simulink model "complementary_filter"  (R2023b)
settings: Solver=FixedStepAuto  StartTime=0.0  StopTime=Tend_slk  FixedStep=Ts_slk  RelTol=1e-3
values from neighbouring files (symbols this model uses):
  acc_pole = 8    [complementary_filter_script.m]    (also in ekf2_script.m = 2)
  alpha = 0.95    [complementary_filter_script.m]
  P0_ps = 100    [complementary_filter_script.m]    (also in ekf1_script.m; ekf2_script.m; ekf3_script.m)
  q_ps = 100e-0    (= 100)    [complementary_filter_script.m]    (also in ekf1_script.m = 200; ekf2_script.m; ekf3_script.m = 170)
  r_ps = 600e+0    (= 600)    [complementary_filter_script.m]    (also in ekf1_script.m = 170; ekf2_script.m; ekf3_script.m = 200)
  Ts_EKF_integr = 0.001    [complementary_filter_script.m]    (also in ekf1_script.m = 0.0001; ekf2_script.m; ekf3_script.m = 0.0001)
  Ts_EKF_meas = 0.01    [complementary_filter_script.m]    (also in ekf1_script.m; ekf2_script.m; ekf3_script.m)
  Ts_meas = 0.01    [complementary_filter_script.m]
  Ts_slk = 0.01    [complementary_filter_script.m]    (also in ekf1_script.m; ekf2_script.m; ekf3_script.m)
  vel_pole = 30    [complementary_filter_script.m]    (also in ekf2_script.m = 20)
  x0_ps = 0    [complementary_filter_script.m]    (also in ekf2_script.m; ekf3_script.m)
settings Model: Creator=teoma  LastModifiedBy=teoma

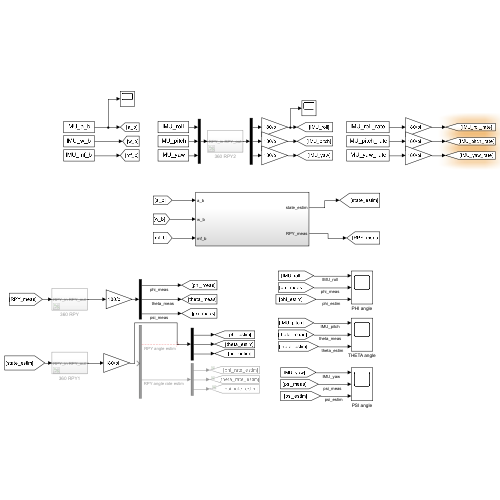
[thumbnail: Simulink's stored preview of the top-level diagram]
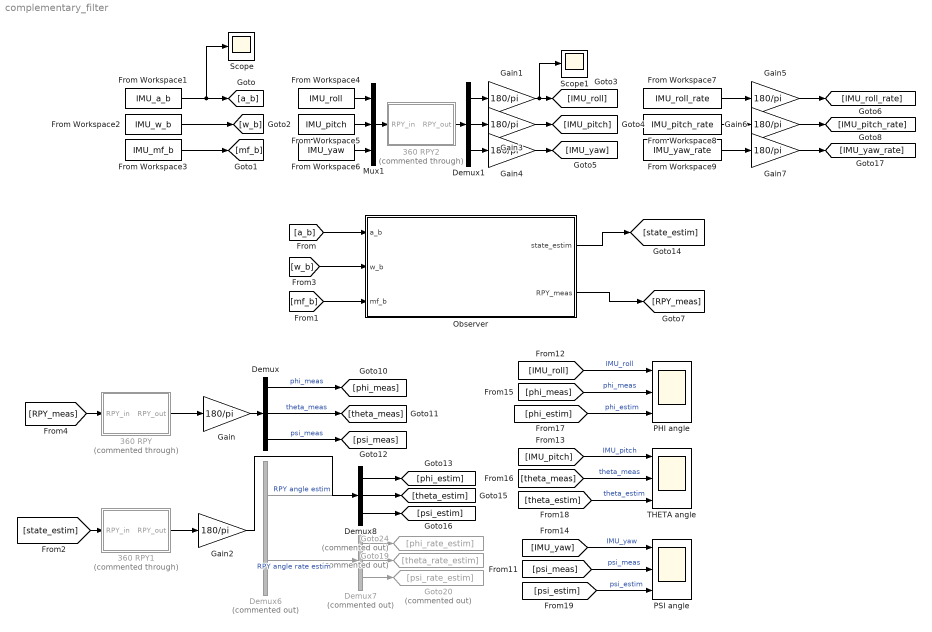
== system complementary_filter ==
  360 RPY : Subsystem  Commented=through
  360 RPY1 : Subsystem  Commented=through
  360 RPY2 : Subsystem  Commented=through
  Demux : Demux  Outputs=3
  Demux1 : Demux  Outputs=3
  Demux6 : Demux  Commented=on  Outputs=2
  Demux7 : Demux  Commented=on  Outputs=3
  Demux8 : Demux  Outputs=3
  From Workspace1 : FromWorkspace  VariableName=IMU_a_b  OutDataTypeStr=double  SampleTime=Ts_slk  Interpolate=off  OutputAfterFinalValue=Setting to zero
  From Workspace2 : FromWorkspace  VariableName=IMU_w_b  OutDataTypeStr=double  SampleTime=Ts_slk  Interpolate=off  OutputAfterFinalValue=Setting to zero
  From Workspace3 : FromWorkspace  VariableName=IMU_mf_b  OutDataTypeStr=double  SampleTime=Ts_slk  Interpolate=off  OutputAfterFinalValue=Setting to zero
  From Workspace4 : FromWorkspace  VariableName=IMU_roll  OutDataTypeStr=double  SampleTime=Ts_slk  Interpolate=off  OutputAfterFinalValue=Setting to zero
  From Workspace5 : FromWorkspace  VariableName=IMU_pitch  OutDataTypeStr=double  SampleTime=Ts_slk  Interpolate=off  OutputAfterFinalValue=Setting to zero
  From Workspace6 : FromWorkspace  VariableName=IMU_yaw  OutDataTypeStr=double  SampleTime=Ts_slk  Interpolate=off  OutputAfterFinalValue=Setting to zero
  From Workspace7 : FromWorkspace  VariableName=IMU_roll_rate  OutDataTypeStr=double  SampleTime=Ts_slk  Interpolate=off  OutputAfterFinalValue=Setting to zero
  From Workspace8 : FromWorkspace  VariableName=IMU_pitch_rate  OutDataTypeStr=double  SampleTime=Ts_slk  Interpolate=off  OutputAfterFinalValue=Setting to zero
  From Workspace9 : FromWorkspace  VariableName=IMU_yaw_rate  OutDataTypeStr=double  SampleTime=Ts_slk  Interpolate=off  OutputAfterFinalValue=Setting to zero
  Gain{,1..7} (8 alike) : Gain  Gain=180/pi
  Goto19 : Goto  Commented=on  GotoTag=theta_rate_estim
  Goto20 : Goto  Commented=on  GotoTag=psi_rate_estim
  Goto24 : Goto  Commented=on  GotoTag=phi_rate_estim
  Mux1 : Mux  Inputs=3
  Observer : Subsystem
  PHI angle : Scope  NumInputPorts=3
  PSI angle : Scope  NumInputPorts=3
  Scope : Scope
  Scope1 : Scope
  THETA angle : Scope  NumInputPorts=3
  wires:
  360 RPY2/1(RPY_out) -> Demux1/1
  From Workspace6/1 -> Mux1/3
  Demux1/3 -> Gain4/1
  Gain3/1 -> [IMU_pitch]
  Demux1/1 -> Gain1/1
  Demux1/2 -> Gain3/1
  From Workspace4/1 -> Mux1/1
  Gain6/1 -> [IMU_pitch_rate]
  From Workspace9/1 -> Gain7/1
  Gain5/1 -> [IMU_roll_rate]
  Mux1/1 -> 360 RPY2/1(RPY_in)
  From Workspace7/1 -> Gain5/1
  From Workspace8/1 -> Gain6/1
  From Workspace1/1 -> [a_b], Scope/1
  Gain1/1 -> Scope1/1, [IMU_roll]
  Gain7/1 -> [IMU_yaw_rate]
  Gain4/1 -> [IMU_yaw]
  From Workspace5/1 -> Mux1/2
  From Workspace3/1 -> [mf_b]
  From Workspace2/1 -> [w_b]
  Demux/2 -> [theta_meas]  "theta_meas"
  Demux7/1 -> Goto24/1
  Demux8/3 -> [psi_estim]
  [state_estim] -> 360 RPY1/1(RPY_in)
  Demux/3 -> [psi_meas]  "psi_meas"
  Demux7/3 -> Goto20/1
  Demux8/2 -> [theta_estim]
  [RPY_meas] -> 360 RPY/1(RPY_in)
  Demux6/1 -> ?  "RPY angle estim"
  [theta_estim] -> THETA angle/3  "theta_estim"
  [psi_estim] -> PSI angle/3  "psi_estim"
  Gain/1 -> Demux/1
  [IMU_pitch] -> THETA angle/1  "IMU_pitch"
  [phi_estim] -> PHI angle/3  "phi_estim"
  Demux/1 -> [phi_meas]  "phi_meas"
  [IMU_roll] -> PHI angle/1  "IMU_roll"
  Demux8/1 -> [phi_estim]
  Demux6/2 -> Demux7/1  "RPY angle rate estim"
  Demux7/2 -> Goto19/1
  Gain2/1 -> Demux8/1
  [psi_meas] -> PSI angle/2  "psi_meas"
  [theta_meas] -> THETA angle/2  "theta_meas"
  360 RPY/1(RPY_out) -> Gain/1
  [IMU_yaw] -> PSI angle/1  "IMU_yaw"
  [phi_meas] -> PHI angle/2  "phi_meas"
  360 RPY1/1(RPY_out) -> Gain2/1
  [mf_b] -> Observer/3(mf_b)
  [a_b] -> Observer/1(a_b)
  Observer/1(state_estim) -> [state_estim]
  Observer/2(RPY_meas) -> [RPY_meas]
  [w_b] -> Observer/2(w_b)

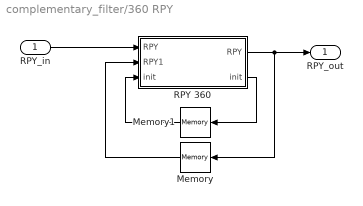
== system complementary_filter/360 RPY ==
  RPY_in : Inport
  Memory : Memory
  Memory1 : Memory
  RPY 360 : MATLAB Function  TreatAsAtomicUnit=on
  RPY_out : Outport
  wires:
  Memory/1 -> RPY 360/2(RPY1)
  Memory1/1 -> RPY 360/3("init ")
  RPY 360/2(init) -> Memory1/1
  RPY 360/1(RPY) -> Memory/1, RPY_out/1
  RPY_in/1 -> RPY 360/1("RPY ")

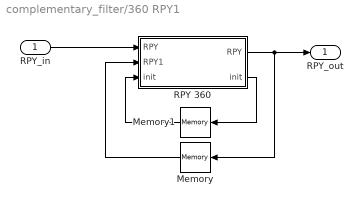
== system complementary_filter/360 RPY1 ==
  RPY_in : Inport
  Memory : Memory
  Memory1 : Memory
  RPY 360 : MATLAB Function  TreatAsAtomicUnit=on
  RPY_out : Outport
  wires:
  Memory/1 -> RPY 360/2(RPY1)
  Memory1/1 -> RPY 360/3("init ")
  RPY 360/2(init) -> Memory1/1
  RPY 360/1(RPY) -> Memory/1, RPY_out/1
  RPY_in/1 -> RPY 360/1("RPY ")

== system complementary_filter/360 RPY2 ==
  RPY_in : Inport
  Memory : Memory
  Memory1 : Memory
  RPY 360 : MATLAB Function  TreatAsAtomicUnit=on
  RPY_out : Outport
  wires:
  Memory/1 -> RPY 360/2(RPY1)
  Memory1/1 -> RPY 360/3("init ")
  RPY 360/2(init) -> Memory1/1
  RPY 360/1(RPY) -> Memory/1, RPY_out/1
  RPY_in/1 -> RPY 360/1("RPY ")

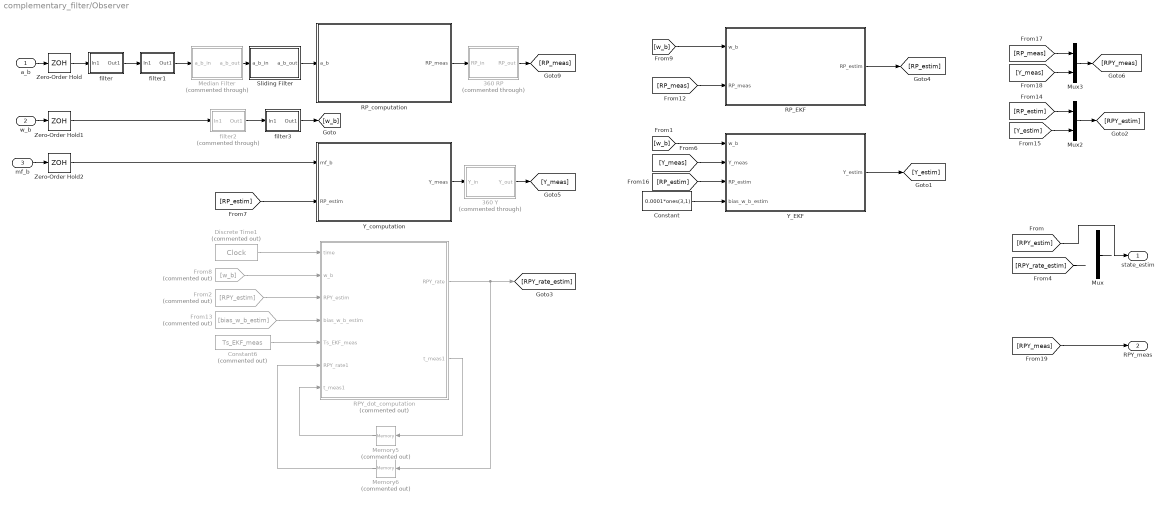
== system complementary_filter/Observer ==
  a_b : Inport
  w_b : Inport  Port=2
  mf_b : Inport  Port=3
  " filter" : Subsystem  mask{p=acc_pole}
      mask prompts: p "pole (p)"
  " filter1" : Subsystem  mask{p=acc_pole}
      mask prompts: p "pole (p)"
  " filter2" : Subsystem  Commented=through  mask{p=5}
      mask prompts: p "pole (p)"
  " filter3" : Subsystem  mask{p=vel_pole}
      mask prompts: p "pole (p)"
  360 RP : Subsystem  Commented=through
  360 Y : Subsystem  Commented=through
  Constant : Constant  Value=0.0001*ones(3,1)
  Constant6 : Constant  Commented=on  Value=Ts_EKF_meas
  Discrete Time1 : DigitalClock  Commented=on  SampleTime=Ts_slk
  From13 : From  Commented=on  GotoTag=bias_w_b_estim
  From2 : From  Commented=on  GotoTag=RPY_estim
  From8 : From  Commented=on  GotoTag=w_b
  Median Filter : Subsystem  Commented=through
  Memory5 : Memory  Commented=on
  Memory6 : Memory  Commented=on
  Mux : Mux  Inputs=2
  Mux2 : Mux  Inputs=2
  Mux3 : Mux  Inputs=2
  RPY_dot_computation : MATLAB Function  Commented=on  TreatAsAtomicUnit=on
  RP_EKF : Subsystem
  RP_computation : MATLAB Function  TreatAsAtomicUnit=on
  Sliding Filter : Subsystem
  Y_EKF : Subsystem
  Y_computation : MATLAB Function  TreatAsAtomicUnit=on
  Zero-Order Hold : ZeroOrderHold  SampleTime=Ts_meas
  Zero-Order Hold1 : ZeroOrderHold  SampleTime=Ts_meas
  Zero-Order Hold2 : ZeroOrderHold  SampleTime=Ts_meas
  state_estim : Outport
  RPY_meas : Outport  Port=2
  wires:
  Memory5/1 -> RPY_dot_computation/7("t_meas1 ")
  Discrete Time1/1 -> RPY_dot_computation/1(time)
  RPY_dot_computation/2(t_meas1) -> Memory5/1
  From8/1 -> RPY_dot_computation/2(w_b)
  Memory6/1 -> RPY_dot_computation/6(RPY_rate1)
  RPY_dot_computation/1(RPY_rate) -> Memory6/1, [RPY_rate_estim]
  Constant6/1 -> RPY_dot_computation/5(Ts_EKF_meas)
  From2/1 -> RPY_dot_computation/3(RPY_estim)
  From13/1 -> RPY_dot_computation/4(bias_w_b_estim)
  [RPY_estim] -> state_estim/1
  [RPY_rate_estim] -> ?
  Mux/1 -> ?
  [RPY_meas] -> RPY_meas/1
  [RP_estim] -> Y_computation/2(RP_estim)
  [Y_meas] -> Y_EKF/2(Y_meas)
  Y_computation/1(Y_meas) -> 360 Y/1(Y_in)
  RP_EKF/1(RP_estim) -> [RP_estim]
  [w_b] -> Y_EKF/1(w_b)
  RP_computation/1(RP_meas) -> 360 RP/1(RP_in)
  [RP_meas] -> RP_EKF/2(RP_meas)
  [w_b] -> RP_EKF/1(w_b)
  Y_EKF/1(Y_estim) -> [Y_estim]
  mf_b/1 -> Zero-Order Hold2/1
  w_b/1 -> Zero-Order Hold1/1
  Constant/1 -> Y_EKF/4(bias_w_b_estim)
  [RP_estim] -> Mux2/1
  [Y_estim] -> Mux2/2
  Mux2/1 -> [RPY_estim]
  [RP_estim] -> Y_EKF/3(RP_estim)
  [RP_meas] -> Mux3/1
  Mux3/1 -> [RPY_meas]
  [Y_meas] -> Mux3/2
  a_b/1 -> Zero-Order Hold/1
  " filter1"/1(Out1) -> Median Filter/1(a_b_in)
  360 Y/1(Y_out) -> [Y_meas]
  " filter"/1(Out1) -> " filter1"/1(In1)
  " filter2"/1(Out1) -> " filter3"/1(In1)
  " filter3"/1(Out1) -> [w_b]
  360 RP/1(RP_out) -> [RP_meas]
  Sliding Filter/1(a_b_out) -> RP_computation/1(a_b)
  Median Filter/1(a_b_out) -> Sliding Filter/1(a_b_in)
  Zero-Order Hold/1 -> " filter"/1(In1)
  Zero-Order Hold1/1 -> " filter2"/1(In1)
  Zero-Order Hold2/1 -> Y_computation/1(mf_b)

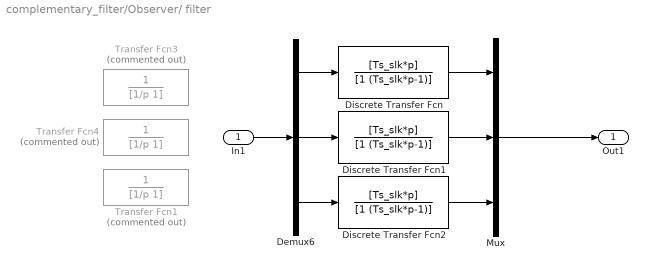
== system complementary_filter/Observer/ filter ==
  In1 : Inport
  Demux6 : Demux  Outputs=3
  Discrete Transfer Fcn : DiscreteTransferFcn  Numerator=[Ts_slk*p]  Denominator=[1 (Ts_slk*p-1)]
  Discrete Transfer Fcn1 : DiscreteTransferFcn  Numerator=[Ts_slk*p]  Denominator=[1 (Ts_slk*p-1)]
  Discrete Transfer Fcn2 : DiscreteTransferFcn  Numerator=[Ts_slk*p]  Denominator=[1 (Ts_slk*p-1)]
  Mux : Mux  Inputs=3
  Transfer Fcn1 : TransferFcn  Commented=on  Denominator=[1/p 1]
  Transfer Fcn3 : TransferFcn  Commented=on  Denominator=[1/p 1]
  Transfer Fcn4 : TransferFcn  Commented=on  Denominator=[1/p 1]
  Out1 : Outport
  wires:
  Discrete Transfer Fcn1/1 -> Mux/2
  Demux6/3 -> Discrete Transfer Fcn2/1
  Mux/1 -> Out1/1
  Discrete Transfer Fcn2/1 -> Mux/3
  Discrete Transfer Fcn/1 -> Mux/1
  In1/1 -> Demux6/1
  Demux6/1 -> Discrete Transfer Fcn/1
  Demux6/2 -> Discrete Transfer Fcn1/1

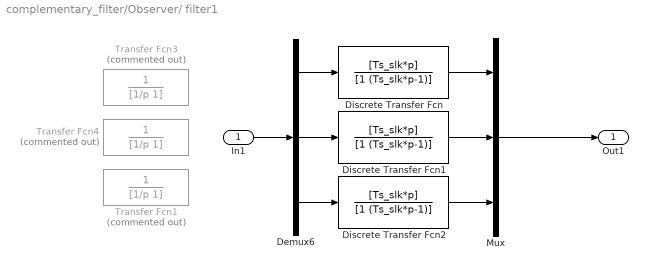
== system complementary_filter/Observer/ filter1 ==
  In1 : Inport
  Demux6 : Demux  Outputs=3
  Discrete Transfer Fcn : DiscreteTransferFcn  Numerator=[Ts_slk*p]  Denominator=[1 (Ts_slk*p-1)]
  Discrete Transfer Fcn1 : DiscreteTransferFcn  Numerator=[Ts_slk*p]  Denominator=[1 (Ts_slk*p-1)]
  Discrete Transfer Fcn2 : DiscreteTransferFcn  Numerator=[Ts_slk*p]  Denominator=[1 (Ts_slk*p-1)]
  Mux : Mux  Inputs=3
  Transfer Fcn1 : TransferFcn  Commented=on  Denominator=[1/p 1]
  Transfer Fcn3 : TransferFcn  Commented=on  Denominator=[1/p 1]
  Transfer Fcn4 : TransferFcn  Commented=on  Denominator=[1/p 1]
  Out1 : Outport
  wires:
  Discrete Transfer Fcn1/1 -> Mux/2
  Demux6/3 -> Discrete Transfer Fcn2/1
  Mux/1 -> Out1/1
  Discrete Transfer Fcn2/1 -> Mux/3
  Discrete Transfer Fcn/1 -> Mux/1
  In1/1 -> Demux6/1
  Demux6/1 -> Discrete Transfer Fcn/1
  Demux6/2 -> Discrete Transfer Fcn1/1

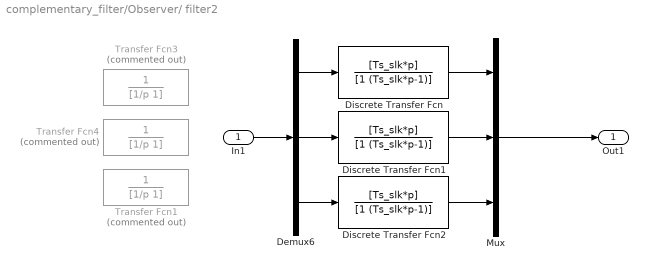
== system complementary_filter/Observer/ filter2 ==
  In1 : Inport
  Demux6 : Demux  Outputs=3
  Discrete Transfer Fcn : DiscreteTransferFcn  Numerator=[Ts_slk*p]  Denominator=[1 (Ts_slk*p-1)]
  Discrete Transfer Fcn1 : DiscreteTransferFcn  Numerator=[Ts_slk*p]  Denominator=[1 (Ts_slk*p-1)]
  Discrete Transfer Fcn2 : DiscreteTransferFcn  Numerator=[Ts_slk*p]  Denominator=[1 (Ts_slk*p-1)]
  Mux : Mux  Inputs=3
  Transfer Fcn1 : TransferFcn  Commented=on  Denominator=[1/p 1]
  Transfer Fcn3 : TransferFcn  Commented=on  Denominator=[1/p 1]
  Transfer Fcn4 : TransferFcn  Commented=on  Denominator=[1/p 1]
  Out1 : Outport
  wires:
  Discrete Transfer Fcn1/1 -> Mux/2
  Demux6/3 -> Discrete Transfer Fcn2/1
  Mux/1 -> Out1/1
  Discrete Transfer Fcn2/1 -> Mux/3
  Discrete Transfer Fcn/1 -> Mux/1
  In1/1 -> Demux6/1
  Demux6/1 -> Discrete Transfer Fcn/1
  Demux6/2 -> Discrete Transfer Fcn1/1

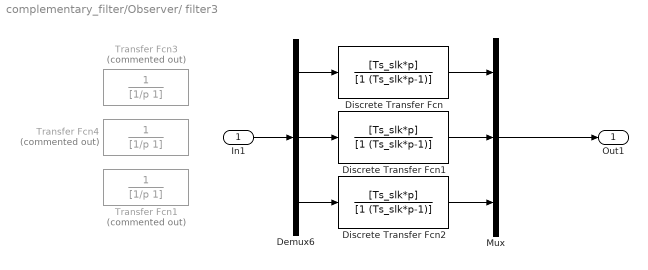
== system complementary_filter/Observer/ filter3 ==
  In1 : Inport
  Demux6 : Demux  Outputs=3
  Discrete Transfer Fcn : DiscreteTransferFcn  Numerator=[Ts_slk*p]  Denominator=[1 (Ts_slk*p-1)]
  Discrete Transfer Fcn1 : DiscreteTransferFcn  Numerator=[Ts_slk*p]  Denominator=[1 (Ts_slk*p-1)]
  Discrete Transfer Fcn2 : DiscreteTransferFcn  Numerator=[Ts_slk*p]  Denominator=[1 (Ts_slk*p-1)]
  Mux : Mux  Inputs=3
  Transfer Fcn1 : TransferFcn  Commented=on  Denominator=[1/p 1]
  Transfer Fcn3 : TransferFcn  Commented=on  Denominator=[1/p 1]
  Transfer Fcn4 : TransferFcn  Commented=on  Denominator=[1/p 1]
  Out1 : Outport
  wires:
  Discrete Transfer Fcn1/1 -> Mux/2
  Demux6/3 -> Discrete Transfer Fcn2/1
  Mux/1 -> Out1/1
  Discrete Transfer Fcn2/1 -> Mux/3
  Discrete Transfer Fcn/1 -> Mux/1
  In1/1 -> Demux6/1
  Demux6/1 -> Discrete Transfer Fcn/1
  Demux6/2 -> Discrete Transfer Fcn1/1

== system complementary_filter/Observer/360 RP ==
  RP_in : Inport
  Memory : Memory
  Memory1 : Memory
  RP 360 : MATLAB Function  TreatAsAtomicUnit=on
  RP_out : Outport
  wires:
  RP_in/1 -> RP 360/1("RP ")
  RP 360/1(RP) -> Memory/1, RP_out/1
  Memory/1 -> RP 360/2(RP1)
  RP 360/2(init) -> Memory1/1
  Memory1/1 -> RP 360/3("init ")

== system complementary_filter/Observer/360 Y ==
  Y_in : Inport
  Memory : Memory
  Memory1 : Memory
  Y 360 : MATLAB Function  TreatAsAtomicUnit=on
  Y_out : Outport
  wires:
  Y_in/1 -> Y 360/1("Y ")
  Y 360/1(Y) -> Memory/1, Y_out/1
  Memory/1 -> Y 360/2(Y1)
  Y 360/2(init) -> Memory1/1
  Memory1/1 -> Y 360/3("init ")

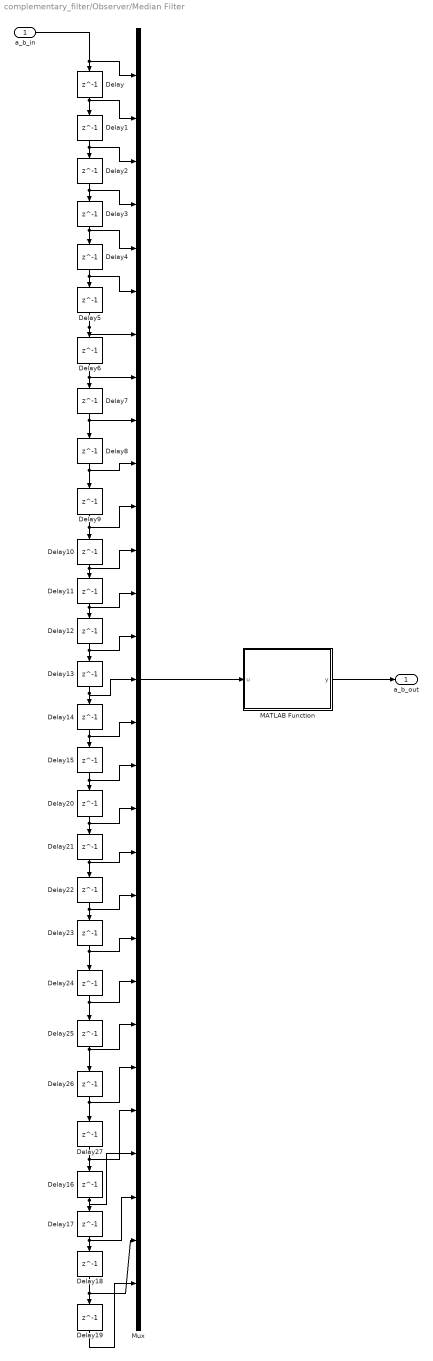
== system complementary_filter/Observer/Median Filter ==
  a_b_in : Inport
  Delay{,1..27} (28 alike) : Delay  DelayLength=1  InitialCondition=zeros(1,3)  SampleTime=Ts_slk
  MATLAB Function : MATLAB Function  TreatAsAtomicUnit=on
  Mux : Mux  Inputs=29
  a_b_out : Outport
  wires:
  a_b_in/1 -> Delay/1, Mux/1
  Delay1/1 -> Delay2/1, Mux/3
  Delay2/1 -> Delay3/1, Mux/4
  Delay/1 -> Delay1/1, Mux/2
  Delay3/1 -> Delay4/1, Mux/5
  Mux/1 -> MATLAB Function/1(u)
  MATLAB Function/1(y) -> a_b_out/1
  Delay4/1 -> Delay5/1, Mux/6
  Delay5/1 -> Delay6/1, Mux/7
  Delay6/1 -> Delay7/1, Mux/8
  Delay8/1 -> Mux/10, Delay9/1
  Delay11/1 -> Mux/13, Delay12/1
  Delay12/1 -> Mux/14, Delay13/1
  Delay7/1 -> Mux/9, Delay8/1
  Delay9/1 -> Delay10/1, Mux/11
  Delay10/1 -> Mux/12, Delay11/1
  Delay13/1 -> Mux/15, Delay14/1
  Delay24/1 -> Mux/22, Delay25/1
  Delay23/1 -> Mux/21, Delay24/1
  Delay20/1 -> Mux/18, Delay21/1
  Delay15/1 -> Mux/17, Delay20/1
  Delay21/1 -> Mux/19, Delay22/1
  Delay27/1 -> Mux/25, Delay16/1
  Delay18/1 -> Delay19/1, Mux/28
  Delay25/1 -> Mux/23, Delay26/1
  Delay22/1 -> Mux/20, Delay23/1
  Delay26/1 -> Mux/24, Delay27/1
  Delay14/1 -> Mux/16, Delay15/1
  Delay17/1 -> Mux/27, Delay18/1
  Delay16/1 -> Mux/26, Delay17/1
  Delay19/1 -> Mux/29

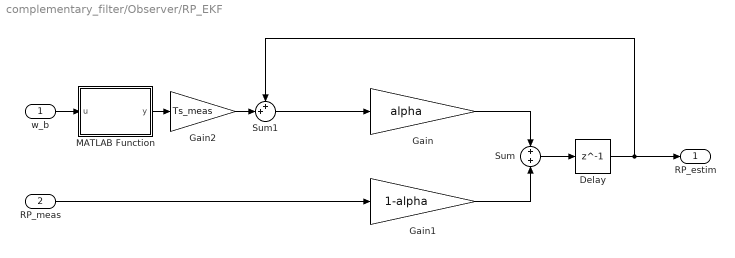
== system complementary_filter/Observer/RP_EKF ==
  w_b : Inport
  RP_meas : Inport  Port=2
  Delay : Delay  DelayLength=1  SampleTime=Ts_meas
  Gain : Gain  Gain=alpha
  Gain1 : Gain  Gain=1-alpha
  Gain2 : Gain  Gain=Ts_meas
  MATLAB Function : MATLAB Function  TreatAsAtomicUnit=on
  Sum : Sum  Inputs=+|+
  Sum1 : Sum  Inputs=++|
  RP_estim : Outport
  wires:
  w_b/1 -> MATLAB Function/1(u)
  RP_meas/1 -> Gain1/1
  MATLAB Function/1(y) -> Gain2/1
  Gain1/1 -> Sum/2
  Gain/1 -> Sum/1
  Sum/1 -> Delay/1
  Sum1/1 -> Gain/1
  Delay/1 -> RP_estim/1, Sum1/1
  Gain2/1 -> Sum1/2

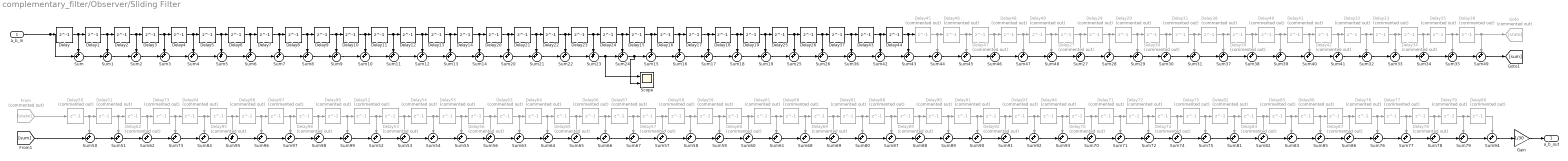
== system complementary_filter/Observer/Sliding Filter ==
  a_b_in : Inport
  Delay{,1..26,37,43..44} (30 alike) : Delay  DelayLength=1  SampleTime=Ts_meas
  Delay{27..36,38..42,45..99} (70 alike) : Delay  Commented=on  DelayLength=1  SampleTime=Ts_slk
  From : From  Commented=on  GotoTag=state
  Gain : Gain  Gain=1/30
  Goto : Goto  Commented=on  GotoTag=state
  Scope : Scope  NumInputPorts=2
  Sum{,1..99} (100 alike) : Sum  Inputs=++|
  a_b_out : Outport
  wires:
  Delay/1 -> Sum/1, Delay1/1
  Delay1/1 -> Sum1/1, Delay2/1
  Delay2/1 -> Sum2/1, Delay3/1
  Delay3/1 -> Sum3/1, Delay4/1
  Sum/1 -> Sum1/2
  Sum1/1 -> Sum2/2
  Sum2/1 -> Sum3/2
  Sum3/1 -> Sum4/2
  Delay4/1 -> Delay5/1, Sum4/1
  Sum4/1 -> Sum5/2
  a_b_in/1 -> Sum/2, Delay/1
  Delay5/1 -> Sum5/1, Delay6/1
  Delay6/1 -> Sum6/1, Delay7/1
  Sum5/1 -> Sum6/2
  Sum6/1 -> Sum7/2
  Sum7/1 -> Sum8/2
  Delay7/1 -> Sum7/1, Delay8/1
  Delay8/1 -> Delay9/1, Sum8/1
  Delay9/1 -> Sum9/1, Delay10/1
  Delay10/1 -> Sum10/1, Delay11/1
  Delay11/1 -> Sum11/1, Delay12/1
  Delay12/1 -> Sum12/1, Delay13/1
  Delay13/1 -> Sum13/1, Delay14/1
  Sum11/1 -> Sum12/2
  Sum12/1 -> Sum13/2
  Sum13/1 -> Sum14/2
  Sum8/1 -> Sum9/2
  Sum9/1 -> Sum10/2
  Sum10/1 -> Sum11/2
  Delay14/1 -> Delay20/1, Sum14/1
  Delay19/1 -> Delay25/1, Sum19/1
  Sum16/1 -> Sum17/2
  Delay15/1 -> Sum15/1, Delay16/1
  Sum24/1 -> Scope/2, Sum15/2
  Sum17/1 -> Sum18/2
  Delay23/1 -> Delay24/1, Sum23/1
  Delay24/1 -> Sum24/1, Delay15/1
  Sum20/1 -> Sum21/2
  Delay22/1 -> Sum22/1, Delay23/1
  Delay18/1 -> Sum18/1, Delay19/1
  Sum23/1 -> Scope/1, Sum24/2
  Sum22/1 -> Sum23/2
  Sum14/1 -> Sum20/2
  Delay20/1 -> Sum20/1, Delay21/1
  Delay17/1 -> Sum17/1, Delay18/1
  Sum18/1 -> Sum19/2
  Delay21/1 -> Sum21/1, Delay22/1
  Delay16/1 -> Sum16/1, Delay17/1
  Sum15/1 -> Sum16/2
  Sum21/1 -> Sum22/2
  Sum41/1 -> Sum32/2
  Delay32/1 -> Sum32/1, Delay33/1
  Sum33/1 -> Sum34/2
  Delay42/1 -> Sum41/1, Delay32/1
  Sum37/1 -> Sum38/2
  Delay41/1 -> Delay42/1, Sum40/1
  Delay31/1 -> Delay38/1, Sum31/1
  Sum28/1 -> Sum29/2
  Delay28/1 -> Sum28/1, Delay29/1
  Delay27/1 -> Sum27/1, Delay28/1
  Delay49/1 -> Sum48/1, Delay27/1
  Sum48/1 -> Sum27/2
  Sum29/1 -> Sum30/2
  Delay48/1 -> Delay49/1, Sum47/1
  Sum44/1 -> Sum45/2
  Delay47/1 -> Sum46/1, Delay48/1
  Delay45/1 -> Sum44/1, Delay46/1
  Delay39/1 -> Sum38/1, Delay40/1
  Sum47/1 -> Sum48/2
  Delay38/1 -> Sum37/1, Delay39/1
  Sum40/1 -> Sum41/2
  Sum46/1 -> Sum47/2
  Sum34/1 -> Sum35/2
  Delay29/1 -> Sum29/1, Delay30/1
  Sum32/1 -> Sum33/2
  Delay40/1 -> Sum39/1, Delay41/1
  Delay46/1 -> Sum45/1, Delay47/1
  Delay33/1 -> Sum33/1, Delay34/1
  Sum27/1 -> Sum28/2
  Delay30/1 -> Sum30/1, Delay31/1
  Sum36/1 -> Sum42/2
  Delay44/1 -> Delay45/1, Sum43/1
  Sum39/1 -> Sum40/2
  Delay37/1 -> Sum36/1, Delay43/1
  Sum26/1 -> Sum36/2
  Sum43/1 -> Sum44/2
  Sum25/1 -> Sum26/2
  Delay35/1 -> Sum35/1, Delay36/1
  Sum42/1 -> Sum43/2
  Delay43/1 -> Sum42/1, Delay44/1
  Sum30/1 -> Sum31/2
  Sum45/1 -> Sum46/2
  Sum31/1 -> Sum37/2
  Delay26/1 -> Sum26/1, Delay37/1
  Delay25/1 -> Sum25/1, Delay26/1
  Delay34/1 -> Sum34/1, Delay35/1
  Sum38/1 -> Sum39/2
  Sum35/1 -> Sum49/2
  Sum19/1 -> Sum25/2
  Delay36/1 -> Goto/1, Sum49/1
  Sum49/1 -> [sum]
  Delay68/1 -> Sum68/1, Delay69/1
  Sum82/1 -> Sum83/2
  Sum68/1 -> Sum69/2
  Sum75/1 -> Sum81/2
  Delay88/1 -> Sum87/1, Delay89/1
  Delay79/1 -> Sum79/1, Delay80/1
  Sum74/1 -> Sum75/2
  Delay69/1 -> Sum69/1, Delay81/1
  Sum90/1 -> Sum91/2
  Sum83/1 -> Sum85/2
  Sum80/1 -> Sum87/2
  Sum88/1 -> Sum89/2
  Sum69/1 -> Sum80/2
  Sum70/1 -> Sum71/2
  Delay78/1 -> Sum78/1, Delay79/1
  Sum92/1 -> Sum93/2
  Sum78/1 -> Sum79/2
  Sum91/1 -> Sum92/2
  Sum85/1 -> Sum86/2
  Sum76/1 -> Sum77/2
  Delay72/1 -> Sum72/1, Delay74/1
  Delay82/1 -> Sum81/1, Delay83/1
  Sum72/1 -> Sum74/2
  Delay94/1 -> Sum93/1, Delay70/1
  Delay85/1 -> Sum83/1, Delay86/1
  Delay74/1 -> Sum74/1, Delay75/1
  Sum93/1 -> Sum70/2
  Delay90/1 -> Sum89/1, Delay91/1
  Delay92/1 -> Sum91/1, Delay93/1
  Delay93/1 -> Delay94/1, Sum92/1
  Delay75/1 -> Delay82/1, Sum75/1
  Sum71/1 -> Sum72/2
  Delay71/1 -> Sum71/1, Delay72/1
  Delay70/1 -> Sum70/1, Delay71/1
  Sum67/1 -> Sum57/2
  Delay57/1 -> Sum57/1, Delay58/1
  Sum58/1 -> Sum59/2
  Sum89/1 -> Sum90/2
  Delay61/1 -> Delay68/1, Sum61/1
  Delay67/1 -> Sum67/1, Delay57/1
  Sum63/1 -> Sum64/2
  Delay66/1 -> Delay67/1, Sum66/1
  Sum94/1 -> Gain/1
  Sum81/1 -> Sum82/2
  Sum77/1 -> Sum78/2
  Delay87/1 -> Sum86/1, Delay76/1
  Delay76/1 -> Sum76/1, Delay77/1
  Delay86/1 -> Delay87/1, Sum85/1
  Sum86/1 -> Sum76/2
  Sum53/1 -> Sum54/2
  Delay53/1 -> Sum53/1, Delay54/1
  Delay56/1 -> Delay63/1, Sum56/1
  Delay52/1 -> Sum52/1, Delay53/1
  Delay99/1 -> Sum99/1, Delay52/1
  Sum99/1 -> Sum52/2
  Sum54/1 -> Sum55/2
  Delay98/1 -> Delay99/1, Sum98/1
  Sum95/1 -> Sum96/2
  Delay97/1 -> Sum97/1, Delay98/1
  Delay95/1 -> Sum95/1, Delay96/1
  Delay55/1 -> Sum55/1, Delay56/1
  Sum98/1 -> Sum99/2
  Sum64/1 -> Sum65/2
  Delay64/1 -> Sum64/1, Delay65/1
  Delay58/1 -> Sum58/1, Delay59/1
  Delay81/1 -> Sum80/1, Delay88/1
  Delay63/1 -> Sum63/1, Delay64/1
  Sum66/1 -> Sum67/2
  Sum97/1 -> Sum98/2
  Delay77/1 -> Sum77/1, Delay78/1
  Sum59/1 -> Sum60/2
  Delay54/1 -> Sum54/1, Delay55/1
  Sum57/1 -> Sum58/2
  Delay89/1 -> Delay90/1, Sum88/1
  Delay65/1 -> Sum65/1, Delay66/1
  Delay96/1 -> Sum96/1, Delay97/1
  Sum52/1 -> Sum53/2
  From/1 -> Delay50/1
  Delay83/1 -> Sum82/1, Delay85/1
  Sum62/1 -> Sum73/2
  Delay84/1 -> Delay95/1, Sum84/1
  Sum65/1 -> Sum66/2
  Sum87/1 -> Sum88/2
  Delay62/1 -> Sum62/1, Delay73/1
  Sum51/1 -> Sum62/2
  Delay91/1 -> Sum90/1, Delay92/1
  Sum84/1 -> Sum95/2
  Sum50/1 -> Sum51/2
  Delay60/1 -> Sum60/1, Delay61/1
  Sum73/1 -> Sum84/2
  Delay73/1 -> Sum73/1, Delay84/1
  Sum55/1 -> Sum56/2
  Sum61/1 -> Sum68/2
  Delay80/1 -> Sum94/1
  Sum96/1 -> Sum97/2
  Sum79/1 -> Sum94/2
  Sum56/1 -> Sum63/2
  Delay51/1 -> Sum51/1, Delay62/1
  Delay50/1 -> Sum50/1, Delay51/1
  Delay59/1 -> Sum59/1, Delay60/1
  Sum60/1 -> Sum61/2
  Gain/1 -> a_b_out/1
  [sum] -> Sum50/2

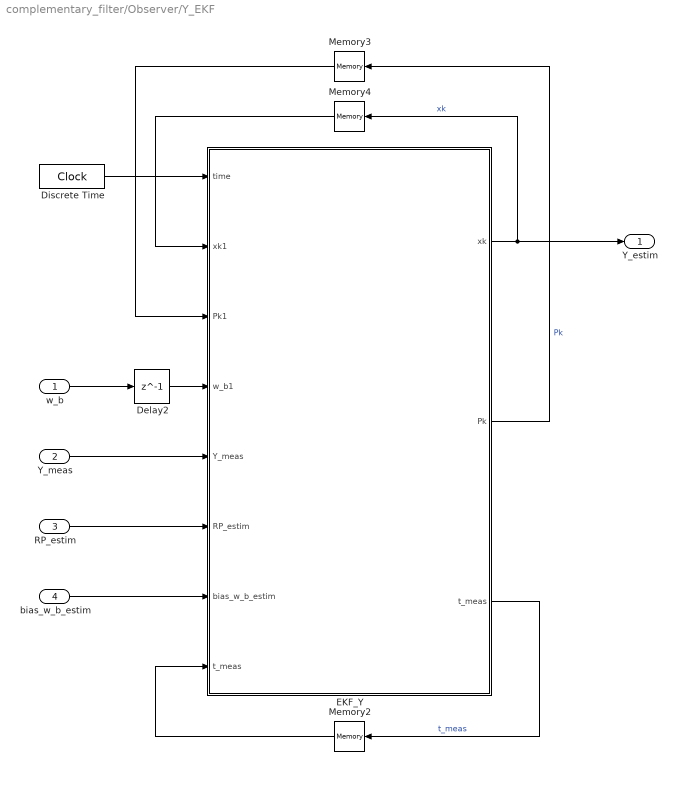
== system complementary_filter/Observer/Y_EKF ==
  w_b : Inport
  Y_meas : Inport  Port=2
  RP_estim : Inport  Port=3
  bias_w_b_estim : Inport  Port=4
  Delay2 : Delay  DelayLength=1  SampleTime=Ts_EKF_meas
  Discrete Time : DigitalClock  SampleTime=Ts_EKF_meas
  EKF_Y : MATLAB Function  TreatAsAtomicUnit=on
  Memory2 : Memory
  Memory3 : Memory  InitialCondition=ones(1,1)*P0_ps
  Memory4 : Memory  InitialCondition=ones(1,1)*x0_ps
  Y_estim : Outport
  wires:
  w_b/1 -> Delay2/1
  EKF_Y/2(Pk) -> Memory3/1  "Pk"
  Memory2/1 -> EKF_Y/8("t_meas ")
  EKF_Y/3(t_meas) -> Memory2/1  "t_meas"
  Y_meas/1 -> EKF_Y/5(Y_meas)
  Discrete Time/1 -> EKF_Y/1(time)
  Memory3/1 -> EKF_Y/3(Pk1)
  Delay2/1 -> EKF_Y/4(w_b1)
  Memory4/1 -> EKF_Y/2(xk1)
  EKF_Y/1(xk) -> Memory4/1, Y_estim/1  "xk"
  bias_w_b_estim/1 -> EKF_Y/7(bias_w_b_estim)
  RP_estim/1 -> EKF_Y/6(RP_estim)

== matlab function complementary_filter/360 RPY/RPY 360 ==
  data: RPY input; RPY output; RPY1 input; init output; init input
function [RPY,init] = RPY_360(RPY,RPY1,init)
if init < 2 
    if init == 0
        init = 1;
        RPY1 = RPY;
    elseif init == 1
        if (RPY - RPY1)'*(RPY - RPY1) > 0.01
            init = 2;
            RPY1 = RPY;
        end
    end
end

% - pi <= PHI <= + pi PHI uses atan2()
if abs(RPY(1) - RPY1(1)) > pi*0.99
    RPY(1) = RPY(1) + sign(RPY1(1))*(2*pi);
end
% - pi/2 <= THETA <= + pi/2 THETA uses asin()
if abs(RPY(2) - RPY1(2)) > pi/2*0.99
    RPY(2) = RPY(2) + sign(RPY1(2))*(2*pi);
end
% - pi <= PSI <= + pi PSI uses atan2()
if abs(RPY(3) - RPY1(3)) > pi*0.99
    RPY(3) = RPY(3) + sign(RPY1(3))*(2*pi);
end
end

== matlab function complementary_filter/Observer/360 Y/Y 360 ==
  data: Y input; Y output; Y1 input; init output; init input
function [Y,init] = Y_360(Y,Y1, init)
if init < 2 
    if init == 0
        init = 1;
        Y1 = Y;
    elseif init == 1
        if (Y - Y1)'*(Y - Y1) > 0.01
            init = 2;
            Y1 = Y;
        end
    end
end

% - pi <= PSI <= + pi PSI uses atan2()
if abs(Y - Y1) > pi*0.99
    Y = Y + sign(Y1)*(2*pi);
end

== matlab function complementary_filter/Observer/360 RP/RP 360 ==
  data: RP input; RP output; RP1 input; init output; init input
function [RP,init] = RP_360(RP,RP1, init)
if init < 2 
    if init == 0
        init = 1;
        RP1 = RP;
    elseif init == 1
        if (RP - RP1)'*(RP - RP1) > 0.01
            init = 2;
            RP1 = RP;
        end
    end
end

% - pi <= PHI <= + pi PHI uses atan2()
if abs(RP(1) - RP1(1)) > pi*0.99
    RP(1) = RP(1) + sign(RP1(1))*(2*pi);
end
% - pi/2 <= THETA <= + pi/2 THETA uses asin()
if abs(RP(2) - RP1(2)) > pi/2*0.99
    RP(2) = RP(2) + sign(RP1(2))*(2*pi);
end

end

== matlab function complementary_filter/Observer/Y_computation ==
  data: mf_b input; RP_estim input; Y_meas output
function Y_meas    = Y_computation(mf_b,RP_estim)
% description:
% - a_b             = measured linear acceleration in body-frame
% - w_b             = measured angular velocity in body-frame
% - mf_b            = measured magnetic field in body-frame
% - mf              = measured magnetic field in body-inertia
% - a_b_disturbe    = linear velocity measurement-noise
% - w_b_disturbe    = angular velocity measurement-noise
% - mf_b_disturbe   = magnetic field measurement-noise

% -------------------------------------------------------------------------------------------
% observation: the following computation works only if the angles
% phi,theta,psy are withing angles (-pi/2,+pi/2) (this is an open set, pi/2 is excluded)
% -------------------------------------------------------------------------------------------

ph_estim = RP_estim(1,1);
th_estim = RP_estim(2,1);

sph = sin(ph_estim);
cph = cos(ph_estim);

sth = sin(th_estim);
cth = cos(th_estim);

ps_meas_num   = mf_b(3)*sph - mf_b(2)*cph;
ps_meas_den = mf_b(1)*cth + mf_b(2)*sth*sph + mf_b(3)*sth*cph;
ps_meas = atan2(ps_meas_num, ps_meas_den);

Y_meas = ps_meas;
end

== matlab function complementary_filter/360 RPY1/RPY 360 ==
  data: RPY input; RPY output; RPY1 input; init output; init input
function [RPY,init] = RPY_360(RPY,RPY1,init)
if init < 2 
    if init == 0
        init = 1;
        RPY1 = RPY;
    elseif init == 1
        if (RPY - RPY1)'*(RPY - RPY1) > 0.01
            init = 2;
            RPY1 = RPY;
        end
    end
end

% - pi <= PHI <= + pi PHI uses atan2()
if abs(RPY(1) - RPY1(1)) > pi*0.99
    RPY(1) = RPY(1) + sign(RPY1(1))*(2*pi);
end
% - pi/2 <= THETA <= + pi/2 THETA uses asin()
if abs(RPY(2) - RPY1(2)) > pi/2*0.99
    RPY(2) = RPY(2) + sign(RPY1(2))*(2*pi);
end
% - pi <= PSI <= + pi PSI uses atan2()
if abs(RPY(3) - RPY1(3)) > pi*0.99
    RPY(3) = RPY(3) + sign(RPY1(3))*(2*pi);
end
end

== matlab function complementary_filter/Observer/Y_EKF/EKF_Y ==
  data: time input; xk1 input size=[1,1]; Pk1 input size=[1,1]; w_b1 input; Y_meas input; RP_estim input; bias_w_b_estim input; t_meas input; q_ps parameter; xk output size=[1,1]; Pk output; t_meas output; r_ps parameter; Ts_EKF_integr parameter; Ts_EKF_meas parameter
function [xk,Pk,t_meas] = EKF_Y(time,xk1,Pk1,w_b1,Y_meas,RP_estim,bias_w_b_estim,t_meas,q_ps,r_ps,Ts_EKF_integr,Ts_EKF_meas)

if time - t_meas >= Ts_EKF_meas
    t_meas = time;
    Q = q_ps;
    R = r_ps;

  % INTEGRATION STEP
    % initial condition
    xt1         =       xk1;                        % initial condition for the state
    Pt1         =       Pk1;                        % initial condition for matrix P

    wp1         =       w_b1(1,1);                  % past value of the p-dir of angular velocity w
    wq1         =       w_b1(2,1);                  % past value of the q-dir of angular velocity w
    wr1         =       w_b1(3,1);                  % past value of the r-dir of angular velocity w

    phi         =       RP_estim(1,1);              % estimate of roll angle (rad)
    theta       =       RP_estim(2,1);              % estimate of pitch angle (rad)  

    bias_wp     =       bias_w_b_estim(1,1);        % estimate of bias of p-dir of angular velocity w
    bias_wq     =       bias_w_b_estim(2,1);        % estimate of bias of q-dir of angular velocity w
    bias_wr     =       bias_w_b_estim(3,1);        % estimate of bias of r-dir of angular velocity w
    % integration loop
    Nstep       = floor(Ts_EKF_meas/Ts_EKF_integr); % number of integration steps to performe in the t_meas time windows
    xt          = zeros(1,1);
    Pt          = zeros(1,1);
    for i = 1:1:Nstep
        % state extraction
            psi         =       xt1(1,1);           % roll angle (rad)
        
            cph         =       cos(phi);
            cth         =       cos(theta);
            cps         =       cos(psi);
            sph         =       sin(phi);
            sth         =       sin(theta);
            sps         =       sin(psi);
            tth         =       sth/cth;
        % integration
            Mf = [0,    sph/cth,    cph/cth,    0,  0,  0;];
            Z1 = [wp1-bias_wp; wq1-bias_wq; wr1-bias_wr; bias_wp; bias_wq; bias_wr;];
            f = Mf*Z1;
            xt = xt1 + Ts_EKF_integr*f;
        
            At1 = 0;
            Pt = Pt1 + Ts_EKF_integr*(At1*Pt1 + Pt1*At1' + Q);
        % house keeping
            xt1 = xt;
            Pt1 = Pt;
    end
  % MEASUREMENT STEP
    Ck = [eye(1)];
    Lk = Pt*Ck'/(Ck*Pt*Ck' + R);
    xk = xt + Lk*(Y_meas - Ck*xt);
    Pk = (eye(1) - Lk*Ck)*Pt;
else
    xk = xk1;
    Pk = Pk1;
end
end

== matlab function complementary_filter/Observer/RP_computation ==
  data: a_b input; RP_meas output
function RP_meas    = RP_computation(a_b)
% description:
% - a_b             = measured linear acceleration in body-frame
% - w_b             = measured angular velocity in body-frame
% - mf_b            = measured magnetic field in body-frame
% - mf              = measured magnetic field in body-inertia
% - a_b_disturbe    = linear velocity measurement-noise
% - w_b_disturbe    = angular velocity measurement-noise
% - mf_b_disturbe   = magnetic field measurement-noise

% -------------------------------------------------------------------------------------------
% observation: the following computation works only if the angles
% phi,theta,psy are withing angles (-pi/2,+pi/2) (this is an open set, pi/2 is excluded)
% -------------------------------------------------------------------------------------------

a_b = -1*a_b;       % need to adjust the sign to use atan2() function correctly

% phi computation
ph_meas = atan2(a_b(2), a_b(3));
sph = sin(ph_meas);
cph = cos(ph_meas);

% theta computation
th_meas = atan2(-a_b(1), (a_b(2)*sph + a_b(3)*cph));

RP_meas = [ph_meas;th_meas];

== matlab function complementary_filter/Observer/RP_EKF/MATLAB Function ==
  data: u input; y output
function y = RPextraction(u)
y = zeros(2,1);
y(1,1) = u(1,1);
y(2,1) = u(2,1);
end

== matlab function complementary_filter/Observer/Median Filter/MATLAB Function ==
  data: u input; y output
function y = fcn(u)
[n,~] = size(u);
n = n/3;
norm = zeros(n,2);
for i = 1:1:n
    u_vect      = u(i*3-2:i*3,1); 
    norm(i,1)   = sqrt(u_vect'*u_vect);     % norm
    norm(i,2)   = i;                        % index
end
for i = 1:n-1
    for j = 1:n-i
        if norm(j,1) > norm(j+1,1)
            % Swap elements
            temp = norm(j,:);
            norm(j,:) = norm(j+1,:);
            norm(j+1,:) = temp;
        end
    end
end
indexMedian = floor(n/2-1);
median = norm(indexMedian,2);
y = u(median*3-2:median*3);
end

== matlab function complementary_filter/360 RPY2/RPY 360 ==
  data: RPY input; RPY output; RPY1 input; init output; init input
function [RPY,init] = RPY_360(RPY,RPY1,init)
if init < 2 
    if init == 0
        init = 1;
        RPY1 = RPY;
    elseif init == 1
        if (RPY - RPY1)'*(RPY - RPY1) > 0.01
            init = 2;
            RPY1 = RPY;
        end
    end
end

% - pi <= PHI <= + pi PHI uses atan2()
if abs(RPY(1) - RPY1(1)) > pi*0.99
    RPY(1) = RPY(1) + sign(RPY1(1))*(2*pi);
end
% - pi/2 <= THETA <= + pi/2 THETA uses asin()
if abs(RPY(2) - RPY1(2)) > pi/2*0.99
    RPY(2) = RPY(2) + sign(RPY1(2))*(2*pi);
end
% - pi <= PSI <= + pi PSI uses atan2()
if abs(RPY(3) - RPY1(3)) > pi*0.99
    RPY(3) = RPY(3) + sign(RPY1(3))*(2*pi);
end
end

== matlab function complementary_filter/Observer/RPY_dot_computation ==
  data: time input; w_b input; RPY_estim input; bias_w_b_estim input; Ts_EKF_meas input; RPY_rate1 input; RPY_rate output; t_meas1 input; t_meas1 output
function [RPY_rate,t_meas1] = RPY_dot_computation(time,w_b,RPY_estim,bias_w_b_estim,Ts_EKF_meas,RPY_rate1,t_meas1)

if time - t_meas1 >= Ts_EKF_meas || time == 0
    wp          =       w_b(1,1);               % p-dir of angular velocity w
    wq          =       w_b(2,1);               % q-dir of angular velocity w
    wr          =       w_b(3,1);               % r-dir of angular velocity w

    phi         =       RPY_estim(1,1);         % roll angle (rad)
    theta       =       RPY_estim(2,1);         % pitch angle (rad)
    psi         =       RPY_estim(3,1);         % yaw angle (rad)  
    bias_wp     =       bias_w_b_estim(1,1)*0;    % bias of p-dir of angular velocity w
    bias_wq     =       bias_w_b_estim(2,1)*0;    % bias of q-dir of angular velocity w
    bias_wr     =       bias_w_b_estim(3,1)*0;   % bias of r-dir of angular velocity w

    cph         =       cos(phi);
    cth         =       cos(theta);
    cps         =       cos(psi);
    sph         =       sin(phi);
    sth         =       sin(theta);
    sps         =       sin(psi);
    tth         =       sth/cth;

    % integration step
    t_meas1 = time;
    W_eta = [1,    sph*tth,    cph*tth;
             0,    cph,        -sph;
             0,    sph/cth,    cph/cth;];
    w_b_corrected = [wp-bias_wp; wq-bias_wq; wr-bias_wr;];
    RPY_rate = W_eta*w_b_corrected;
else
    RPY_rate = RPY_rate1;
end
end
